simulink model "TB_6DOF_v1"  (R2026a)
settings: Solver=ode45  MaxStep=0.001
PreLoadFcn:
  | mc_inputs
settings Model: Creator=aditi  LastModifiedBy=aditi

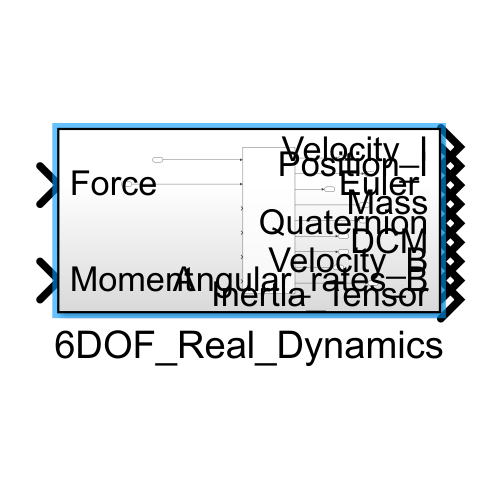
[thumbnail: Simulink's stored preview of the top-level diagram]
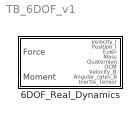
== system TB_6DOF_v1 ==
  6DOF_Real_Dynamics : Subsystem

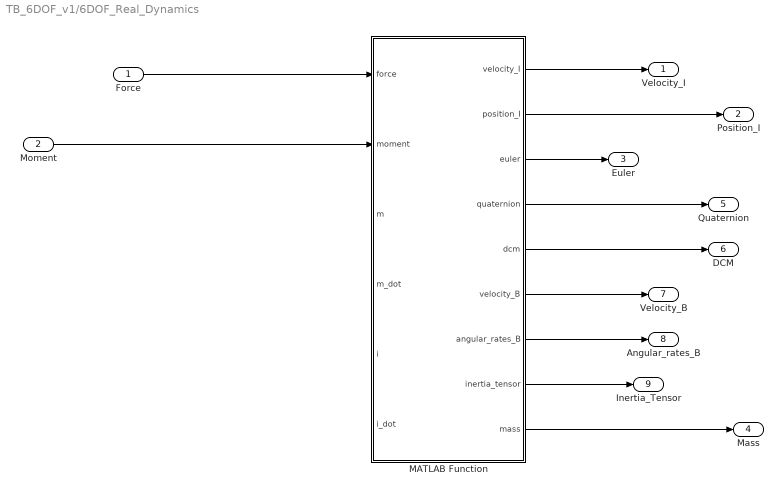
== system TB_6DOF_v1/6DOF_Real_Dynamics ==
  Force : Inport
  Moment : Inport  Port=2
  MATLAB Function : MATLAB Function  TreatAsAtomicUnit=on
  Velocity_I : Outport
  Position_I : Outport  Port=2
  "Euler " : Outport  Port=3
  Mass : Outport  Port=4
  Quaternion : Outport  Port=5
  DCM : Outport  Port=6
  Velocity_B : Outport  Port=7
  Angular_rates_B : Outport  Port=8
  Inertia_Tensor : Outport  Port=9
  wires:
  Moment/1 -> MATLAB Function/2(moment)
  Force/1 -> MATLAB Function/1(force)
  MATLAB Function/1(velocity_I) -> Velocity_I/1
  MATLAB Function/2(position_I) -> Position_I/1
  MATLAB Function/4(quaternion) -> Quaternion/1
  MATLAB Function/3(euler) -> "Euler "/1
  MATLAB Function/5(dcm) -> DCM/1
  MATLAB Function/6(velocity_B) -> Velocity_B/1
  MATLAB Function/7(angular_rates_B) -> Angular_rates_B/1
  MATLAB Function/8(inertia_tensor) -> Inertia_Tensor/1
  MATLAB Function/9(mass) -> Mass/1

== matlab function TB_6DOF_v1/6DOF_Real_Dynamics/MATLAB Function ==
  data: velocity_I output; force input; moment input; position_I output; euler output; quaternion output; dcm output; velocity_B output; angular_rates_B output; inertia_tensor output; mass output; m input; m_dot input; i input; i_dot input
function [velocity_I, position_I, euler, quaternion, dcm, velocity_B, angular_rates_B, inertia_tensor, mass] = custom_aerospace_6dof(force, moment, m, m_dot, i, i_dot)
    % =====================================================================
    % ALL 9 OUTPUTS DERIVED DIRECTLY FROM FIRST-PRINCIPLES PHYSICS
    % =====================================================================
    
    %% 1. TIME STEP PARAMETER
    dt = 0.01;                 % Time step size (seconds)
    
    %% 2. PERSISTENT STATE MEMORY (Kinematics only)
    persistent v_b_state omega_b_state q_state P_i_state
    
    if isempty(v_b_state)
        v_b_state     = [0;0;0];   % Initial Body Velocity [u; v; w]
        omega_b_state = [0;0;0];   % Initial Body Angular Rates [p; q; r]
        q_state       = [1;0;0;0]; % Initial Quaternion (Aligned with ground)
        P_i_state     = [0;0;0];   % Initial Inertial Position [x; y; z]
    end
    
    %% 3. MASS & INERTIA TENSOR CALCULATION
    % Map input mass directly to output
    mass = m; 
    
    % Calculate shifting Center of Gravity displacement [xd; yd; zd]
    % (Assuming initial reference mass m_initial can be tracked or relative change used)
    persistent m_initial;
    if isempty(m_initial)
        m_initial = m;
    end
    x_d = 0.05 * (m_initial - mass); 
    
    % Apply input Inertia (I) and Inertia Derivative (I_dot) with Parallel Axis Theorem
    inertia_tensor = i - mass * [0,    0,    0;
                                  0,  x_d^2,  0;
                                  0,    0,  x_d^2];
                                  
    %% 4. ROTATIONAL DYNAMICS (Angular Rates)
    % Derived via Euler's Rotational Equations + Variable Inertia Correction
    omega_b_dot = inertia_tensor \ (moment - cross(omega_b_state, inertia_tensor * omega_b_state) - i_dot * omega_b_state);
    omega_b_state = omega_b_state + omega_b_dot * dt;
    angular_rates_B = omega_b_state; % Map to output
    
    %% 5. TRANSLATIONAL DYNAMICS (Body Velocity)
    % Derived via Newton's Second Law + Coriolis/Transport Theorem
    v_b_dot = (force / mass) - (m_dot / mass) * v_b_state - cross(angular_rates_B, v_b_state);
    v_b_state = v_b_state + v_b_dot * dt;
    velocity_B = v_b_state; % Map to output
    
    %% 6. ORIENTATION KINEMATICS (Quaternion & DCM)
    p = angular_rates_B(1); q_val = angular_rates_B(2); r = angular_rates_B(3);
    omega_q = [0,    -p, -q_val, -r;
               p,     0,    r, -q_val;
               q_val, -r,    0,    p;
               r,  q_val,   -p,    0];
    q_dot = 0.5 * omega_q * q_state;
    
    % Integrate and strictly normalize to prevent numerical axis warping
    q_state = q_state + q_dot * dt;
    q_state = q_state / norm(q_state);
    quaternion = q_state; % Map to output 
    
    % Construct DCM directly from Quaternion components (Rodrigues derivation)
    q0 = quaternion(1); q1 = quaternion(2); q2 = quaternion(3); q3 = quaternion(4);
    dcm = [1 - 2*(q2^2 + q3^2),   2*(q1*q2 - q0*q3),   2*(q1*q3 + q0*q2);
           2*(q1*q2 + q0*q3), 1 - 2*(q1^2 + q3^2),   2*(q2*q3 - q0*q1);
           2*(q1*q3 - q0*q2), 2*(q2*q3 + q0*q1), 1 - 2*(q1^2 + q2^2)];
           
    %% 7. BRIDGING KINEMATICS TO INERTIAL SPACE (Inertial Velocity & Position)
    velocity_I = dcm * velocity_B; 
    
    P_i_state = P_i_state + velocity_I * dt;
    position_I = P_i_state; % Map to output
    
    %% 8. EULER ANGLES EXTRACTION
    phi   = atan2(dcm(3,2), dcm(3,3));     % Roll
    theta = -asin(dcm(3,1));              % Pitch
    psi   = atan2(dcm(2,1), dcm(1,1));     % Yaw
    euler = [phi; theta; psi];            % Map to output
end
